simulink model "simulink_template_2_3"  (R2025b)
settings: Solver=ode4  StartTime=0.0  StopTime=10.0  FixedStep=1e-3  RelTol=1e-3
values from neighbouring files (symbols this model uses):
  a = vc/Ta    (= 0.333333333333)    [fcn.m]    (also in part2.m = [xf,xi,kf*cos(thetaf)-3*xf, ki*cos(thetai)+3*xi ])
  b = [yf,yi,kf*sin(thetaf)-3*yf, ki*sin(thetai)+3*yi ]    [part2.m]
  qi = [-1; -1; pi/2]    [EX_opt_2_leo.m]    (also in part2.m = [xi;yi;thetai]; script_2_motion_planning.m)
settings Model: Creator=alber  LastModifiedBy=llp
settings RTWCC: GPUComputeCapability=3.5

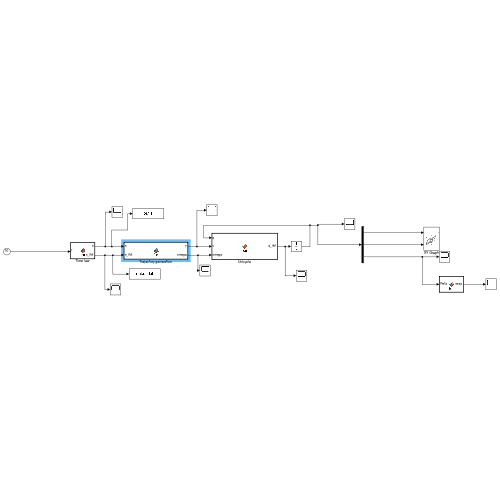
[thumbnail: Simulink's stored preview of the top-level diagram]
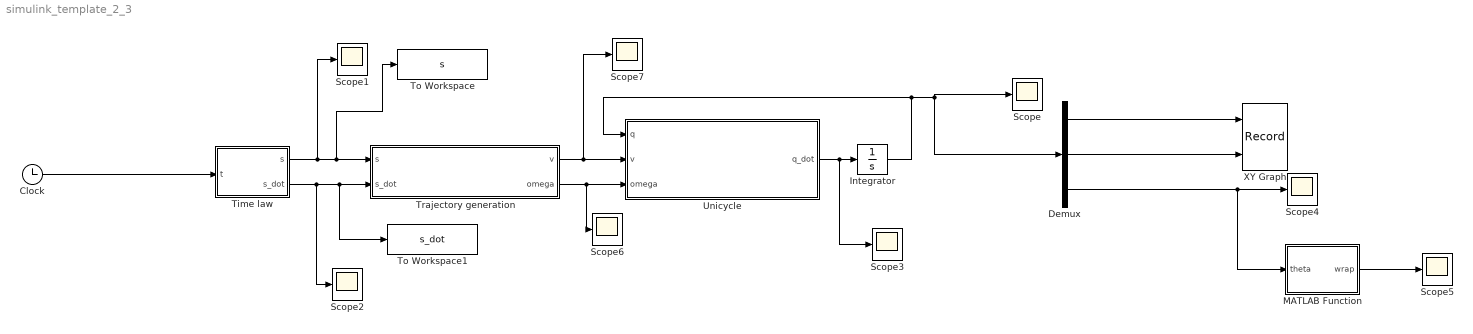
== system simulink_template_2_3 ==
  Clock : Clock
  Demux : Demux  Outputs=3
  Integrator : Integrator  InitialCondition=qi
  MATLAB Function : MATLAB Function  TreatAsAtomicUnit=on
  Scope{,1..7} (8 alike) : Scope
      Scope settings: ActiveDisplayYMinimum=-5.1633659830951473  ActiveDisplayYMaximum=7.498388194097334
      Scope1 settings: ActiveDisplayYMinimum=-0.12499999999999997  ActiveDisplayYMaximum=1.125
      Scope2 settings: ActiveDisplayYMinimum=-0.024999999999999994  ActiveDisplayYMaximum=0.225  DataLoggingVariableName=ScopeData2
      Scope3 settings: ActiveDisplayYMinimum=-1  ActiveDisplayYMaximum=1  DataLoggingVariableName=ScopeData3
      Scope4 settings: ActiveDisplayYMinimum=-1  ActiveDisplayYMaximum=1  DataLoggingVariableName=ScopeData5
      Scope5 settings: ActiveDisplayYMinimum=-1  ActiveDisplayYMaximum=1  DataLoggingVariableName=ScopeData4
      Scope6 settings: ActiveDisplayYMinimum=-0.33870492786676076  ActiveDisplayYMaximum=3.0483443508008472  DataLoggingVariableName=ScopeData6
      Scope7 settings: ActiveDisplayYMinimum=-0.10252982019566476  ActiveDisplayYMaximum=0.92276838176098308  DataLoggingVariableName=ScopeData7
  Time law : MATLAB Function  TreatAsAtomicUnit=on
  To Workspace : ToWorkspace  VariableName=s  SaveFormat=Timeseries  SampleTime=-1
  To Workspace1 : ToWorkspace  VariableName=s_dot  SaveFormat=Timeseries  SampleTime=-1
  Trajectory generation : MATLAB Function  TreatAsAtomicUnit=on
  Unicycle : MATLAB Function  TreatAsAtomicUnit=on
  XY Graph : Record  NumPorts=2.0  FileSettingsInternal="{\"entries\":[{\"content\":{\"excelSettings\":{\"content\":{},\"type\":\"Streamout.ExcelSettings\"},\"parquetSettings\":{\"content\":{},\"type\":\"Streamout.ParquetSettings\"}},\"type\":\"Streamout.FileSettingStorage\",\"uuid\":\"\"}],\"packageUris\":[\"http:\\/\\/schema.mathworks.com\\/mf0\\/streamout_blocks\\/R2020a\"],\"version\":\"1.0\"}"  FrameSettings=[0, 0]  Layout=[1 1]  SignalsInternal="{\"entries\":[{\"content\":{\"signals\":[{\"content\":{\"blockPath\":[],\"dimensions\":[1,1],\"domain\":\"\",\"lineColor\":\"#a2142f\",\"plots\":[ 1 ],\"port\":1,\"sid\":[\"\"],\"signalID\":1,\"signalName\":\"Demux:1\"},\"type\":\"RecordBlkView.Signal\",\"uuid\":\"\"},{\"content\":{\"blockPath\":[],\"dimensions\":[1,1],\"domain\":\"\",\"lineColor\":\"#139fff\",\"plots\":[ 1 ],\"port\":2,\"sid\":[\"\"],\"signalID\":2,\"signalName\":\"Demux:2\"},\"type\":\"RecordBlkView.Signal\",\"uuid\":\"\"}]},\"type\":\"RecordBlkView.InputSignals\",\"uuid\":\"\"}],\"packageUris\":[\"http:\\/\\/schema.mathworks.com\\/mf0\\/streamout_blocks\\/R2020a\"],\"version\":\"1.0\"}"  VisualizationBindings="{\"xyplotplugin\":{\"info\":[{\"series\":[{\"bindingParametersList\":[{\"parameter\":\"X-Axis\",\"signalID\":1,\"signalName\":\"Demux:1\"},{\"parameter\":\"Y-Axis\",\"signalID\":2,\"signalName\":\"Demux:2\"}],\"seriesID\":0}],\"subplotID\":1}]}}"  CompatibilityTag=XY
  wires:
  Clock/1 -> Time law/1(t)
  Time law/1(s) -> Scope1/1, To Workspace/1, Trajectory generation/1(s)
  Time law/2(s_dot) -> Scope2/1, To Workspace1/1, Trajectory generation/2(s_dot)
  Trajectory generation/1(v) -> Scope7/1, Unicycle/2(v)
  Trajectory generation/2(omega) -> Scope6/1, Unicycle/3(omega)
  Unicycle/1(q_dot) -> Scope3/1, Integrator/1
  Demux/1 -> XY Graph/1
  Integrator/1 -> Demux/1, Scope/1, Unicycle/1(q)
  MATLAB Function/1(wrap) -> Scope5/1
  Demux/2 -> XY Graph/2
  Demux/3 -> MATLAB Function/1(theta), Scope4/1

== matlab function simulink_template_2_3/Trajectory generation ==
  data: v output; s input; s_dot input; omega output; a parameter; b parameter
function [v, omega] = fcn(s, s_dot, a, b)
    % 1. Calcolo delle derivate spaziali prime (x' e y')
    % Basate sul polinomio cubico: y1(s) = a1*s^3 - a2*(s-1)^3 + a3*s^2*(s-1) + a4*s*(s-1)^2
    x_p = 3*a(1)*s^2 - a(2)*(3*s^2 - 6*s + 3) + a(3)*(3*s^2 - 2*s) + a(4)*(3*s^2 - 4*s + 1);
    y_p = 3*b(1)*s^2 - b(2)*(3*s^2 - 6*s + 3) + b(3)*(3*s^2 - 2*s) + b(4)*(3*s^2 - 4*s + 1);
    
    % 2. Calcolo delle derivate spaziali seconde (x'' e y'')
    x_pp = 6*a(1)*s - a(2)*(6*s - 6) + a(3)*(6*s - 2) + a(4)*(6*s - 4);
    y_pp = 6*b(1)*s - b(2)*(6*s - 6) + b(3)*(6*s - 2) + b(4)*(6*s - 4);
    
    % 3. Ingressi geometrici (tilde) assumendo marcia in avanti (k=0)
    v_tilde = sqrt(x_p^2 + y_p^2);
    
    % NOTA: Aggiungo 'eps' (un numero minuscolo) al denominatore per evitare 
    % che Simulink vada in crash per divisione per zero se il robot è fermo.
    omega_tilde = (x_p * y_pp - y_p * x_pp) / (x_p^2 + y_p^2 + eps);
    
    % 4. Ingressi fisici nel tempo (Moltiplicazione per s_dot)
    v = v_tilde * s_dot;
    omega = omega_tilde * s_dot;
end

== matlab function simulink_template_2_3/Time law ==
  data: t input; s output; s_dot output
function [s, s_dot] = fcn(t)

Ta = 2;
Tc = 3;

T1 = Ta;
T2 = Ta + Tc;
T3 = 2*Ta + Tc;

vc = 1/(Ta+Tc);
acc = vc/Ta;


% velocità
if t < T1
    s = 0.5*acc*t^2;
    s_dot = acc*t;

elseif t < T2
    s = 0.5*acc*Ta^2 + vc*(t - Ta);
    s_dot = vc;

elseif t < T3
    s = 0.5*acc*Ta^2 + vc*Tc + vc*(t - Ta - Tc)- 0.5*acc*(t - Ta - Tc)^2;
    s_dot = vc - acc*(t - Ta - Tc);

else
    s = 1;
    s_dot = 0;
end

== matlab function simulink_template_2_3/Unicycle ==
  data: q_dot output; q input; v input; omega input
function q_dot = fcn(q, v, omega)
%write the unicycle model
q_dot= zeros(3,1);

q_dot(1) = v*cos(q(3));
q_dot(2) = v*sin(q(3));
q_dot(3) = omega;

== matlab function simulink_template_2_3/MATLAB Function ==
  data: theta input; wrap output
function wrap = fcn(theta)

wrap = mod(theta+pi,2*pi)-pi ;
